simulink model "stopafterdistance"  (R2016a)
settings: Solver=FixedStepAuto  StartTime=0.0  StopTime=inf  RelTol=1e-3
model workspace (MAT data in the model file):
  SL_ROS_VariableLengthArrays_MaxSizes.CommonInfo.ArrayTruncateAction = 'EmitWarning'
  SL_ROS_VariableLengthArrays_MaxSizes.MsgTypeMap = containers.Map
  SL_ROS_VariableLengthArrays_MaxSizes.MsgTypeMap.serialization.keys = {'sensor_msgs/LaserScan'}
  SL_ROS_VariableLengthArrays_MaxSizes.MsgTypeMap.serialization.values{1}(1).PropertyName = 'Ranges'
  SL_ROS_VariableLengthArrays_MaxSizes.MsgTypeMap.serialization.values{1}(1).DataType = 'single'
  SL_ROS_VariableLengthArrays_MaxSizes.MsgTypeMap.serialization.values{1}(1).MaxLength = 180
  SL_ROS_VariableLengthArrays_MaxSizes.MsgTypeMap.serialization.values{1}(2).PropertyName = 'Intensities'
  SL_ROS_VariableLengthArrays_MaxSizes.MsgTypeMap.serialization.values{1}(2).DataType = 'single'
  SL_ROS_VariableLengthArrays_MaxSizes.MsgTypeMap.serialization.values{1}(2).MaxLength = 180
  SL_ROS_VariableLengthArrays_MaxSizes.MsgTypeMap.serialization.uniformity = 0
  SL_ROS_VariableLengthArrays_MaxSizes.MsgTypeMap.serialization.keyType = 'char'
  SL_ROS_VariableLengthArrays_MaxSizes.MsgTypeMap.serialization.valueType = 'any'
libraries: robotlib x3
settings Model: Creator=sprinkle  LastModifiedBy=ece446
settings OptimizationCC: OptimizeModelRefInitCode=on  LifeSpan=Inf  MaxStackSize=64
settings HardwareCC: ProdBitPerPointer=32  ProdLargestAtomicFloat=None  ProdIntDivRoundTo=Undefined  ProdEndianess=Unspecified  ProdWordSize=32  ProdHWDeviceType=Generic->Unspecified (assume 32-bit Generic)
settings RTWCC: SystemTargetFile=ert.tlc  HardwareBoard=Robot Operating System (ROS)  TemplateMakefile=ert_default_tmf  GenerateReport=on  Toolchain=Catkin  IncludeHyperlinkInReport=on  LaunchReport=on  TargetLang=C++  GenerateTraceInfo=on  GenerateTraceReport=on  GenerateTraceReportSl=on  GenerateTraceReportSf=on  GenerateTraceReportEml=on
settings CodeAppCC: ForceParamTrailComments=on  IgnoreCustomStorageClasses=off  OperatorAnnotations=on  SimulinkDataObjDesc=on  SFDataObjDesc=on  MATLABFcnDesc=on  InsertBlockDesc=on  MATLABSourceComments=on

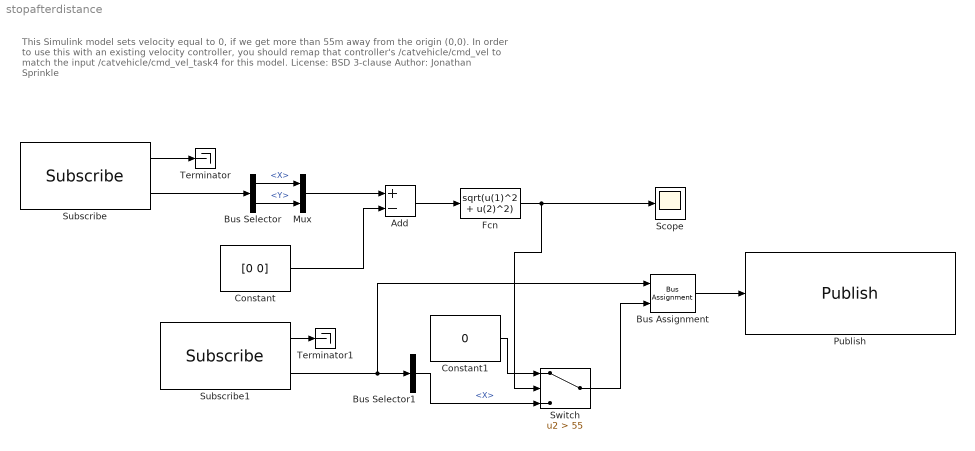
== system stopafterdistance ==
  note: This Simulink model sets velocity equal to 0, if we get more than 55m away from the origin (0,0). In order to use this with an existing velocity controller, you should remap that controller's /catvehicle/cmd_vel to match the input /catvehicle/cmd_vel_task4 for this model.
      |
      | License: BSD 3-clause
      | Author: Jonathan Sprinkle
  Add : Sum  Inputs=+-
  Bus Assignment : BusAssignment  AssignedSignals=Linear.X
  Bus Selector : BusSelector  OutputSignals=Pose.Pose.Position.X,Pose.Pose.Position.Y
  Bus Selector1 : BusSelector  OutputSignals=Linear.X
  Constant : Constant  Value=[0 0]
  Constant1 : Constant  Value=0
  Fcn : Fcn  Expr=sqrt(u(1)^2 + u(2)^2)
  Mux : Mux  Inputs=2
  Publish : robotlib/Publish  SourceLibraryInfo=This block requires Robotics System Toolbox  topicSource=Specify your own  topic=/catvehicle/cmd_vel  messageType=geometry_msgs/Twist  messageQueueLength=1
  Scope : Scope
  Subscribe : robotlib/Subscribe  SourceLibraryInfo=This block requires Robotics System Toolbox  topicSource=Select from ROS network  topic=/catvehicle/odom  messageType=nav_msgs/Odometry  sampleTime=-1  messageQueueLength=1
  Subscribe1 : robotlib/Subscribe  SourceLibraryInfo=This block requires Robotics System Toolbox  topicSource=Specify your own  topic=/catvehicle/cmd_vel_task4  messageType=geometry_msgs/Twist  sampleTime=-1  messageQueueLength=1
  Switch : Switch  Criteria=u2 > Threshold  Threshold=55
  Terminator : Terminator
  Terminator1 : Terminator
  wires:
  Subscribe/1 -> Terminator/1
  Subscribe/2 -> Bus Selector/1
  Bus Selector/1 -> Mux/1  "<X>"
  Bus Selector/2 -> Mux/2  "<Y>"
  Mux/1 -> Add/1
  Constant/1 -> Add/2
  Add/1 -> Fcn/1
  Fcn/1 -> Switch/2, Scope/1
  Subscribe1/1 -> Terminator1/1
  Subscribe1/2 -> Bus Assignment/1, Bus Selector1/1
  Switch/1 -> Bus Assignment/2
  Bus Selector1/1 -> Switch/3  "<X>"
  Bus Assignment/1 -> Publish/1
  Constant1/1 -> Switch/1
